simulink model "VSCHVDCunitblackstart"  (R2025b)
settings: Solver=VariableStepAuto  StartTime=0  StopTime=25  FixedStep=5e-5  RelTol=1e-3
PreLoadFcn:
  | HVDCParameters;
  | BlackStartMMCParameters;
undefined symbols (not defined in the file): DiscIntNeverNeededParam, FRated, frt, gGFM, grid, Lbase, Lr, Lt, lvrt, mGFM, mpptOmega, mpptWindSpeed, Nm, pmsm, PRated, Rc, rpir, Rr, Rt, time, Tpir, Ts, Vbase, Vdcs0, VRated, Vt2, windController, windTurbine, Zbase
libraries: fl_lib x47, ee_lib x41, nesl_utility x33, eeGeneralControl x13, eeTransforms x12, slpidlib x8, eeSinusoidalMeasurementV2 x4, simulink x2, eeSinusoidalMeasurement x1, eeStairGenerator x1
(part 1 of 5)
settings Model: SimulationMode=accelerator  Creator=Rajarshi  LastModifiedBy=rajarshd
settings SolverCC: ZeroCrossControl=DisableAll  ZeroCrossAlgorithm=Adaptive  AutoInsertRateTranBlk=on
settings DataIOCC: InitialState=xFinal  SaveFormat=StructureWithTime  SaveOutput=off  DSMLogging=off  StreamToWks=off  SaveTime=off  ReturnWorkspaceOutputsName=blackstartResults
settings DebuggingCC: InheritedTsInSrcMsg=none
settings ModelReferenceCC: PropagateSignalLabelsOutOfModel=off
settings SimscapeCC: SimscapeNormalizeSystem=off

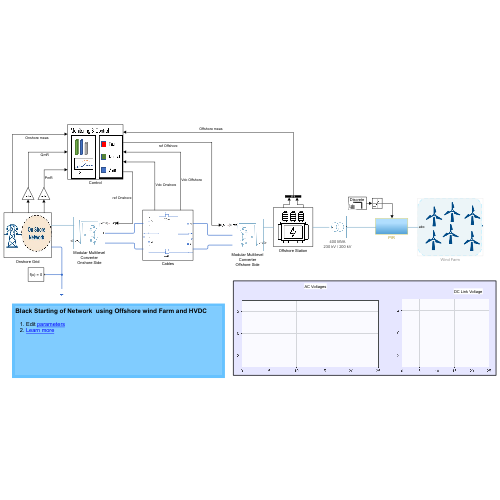
[thumbnail: Simulink's stored preview of the top-level diagram]
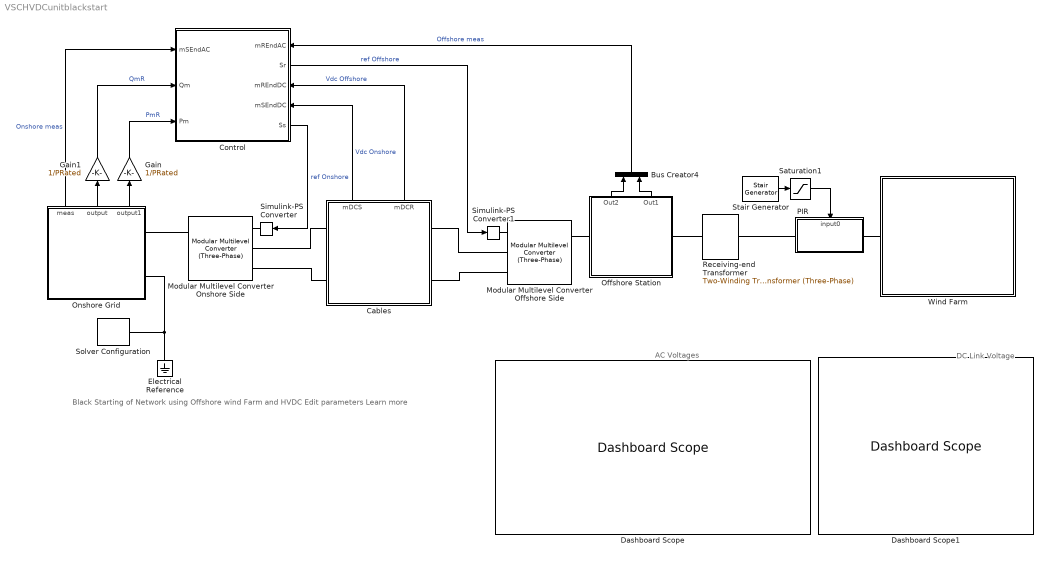
== system VSCHVDCunitblackstart ==
  note: DC Link Voltage
  note: AC Voltages
  note: Black Starting of Network using Offshore wind Farm and HVDC
      |
      | Edit parameters
      | Learn more
  Bus Creator4 : BusCreator  Inputs=2
  Cables : Subsystem
      settings: PortSchema="{\"entries\":[{\"content\":{\"sides\":[{\"content\":{\"connectorIds\":[\"LConn1\",\"LConn2\"]},\"type\":\"ConnectorPlacement.EquallySpacedRectSide\",\"uuid\":\"66d4cfbf-dcba-4749-bf5d-5811a775276e\"},{\"content\":{\"connectorIds\":[\"RConn1\",\"RConn2\"],\"side\":\"RIGHT\"},\"type\":\"ConnectorPlacement.EquallySpacedRectSide\",\"uuid\":\"35abdffa-cda0-46f2-9903-3f86a9532248\"},{\"content\":{\"connectorIds\":[\"Out1\",\"Out2\"],\"side\":\"TOP\"},\"type\":\"ConnectorPlacement.EquallySpacedRectSide\",\"uuid\":\"3c5502e5-1b76-444d-b26b-a5789383a319\"}]},\"type\":\"ConnectorPlacement.EquallySpacedConnector\",\"uuid\":\"b78b2c4f-7eb3-43f3-aa61-891430661a3a\"}],\"packageUris\":[\"http://schema.mathworks.com/mf0/Connector/R2020b\"],\"version\":\"1.0\"}"
      mask Display: image('HVDCCable.PNG');
  Control : Subsystem
      settings: PortSchema="{\"entries\":[{\"content\":{\"sides\":[{\"content\":{\"connectorIds\":[\"In1\",\"In2\",\"In3\"]},\"type\":\"ConnectorPlacement.EquallySpacedRectSide\",\"uuid\":\"2efe798b-3041-46d6-be94-ed23c5e86f39\"},{\"content\":{\"connectorIds\":[\"In4\",\"Out1\",\"In5\",\"In6\",\"Out2\"],\"side\":\"RIGHT\"},\"type\":\"ConnectorPlacement.EquallySpacedRectSide\",\"uuid\":\"10311844-b4ae-4332-a927-ed09106eeb00\"},{\"content\":{\"side\":\"TOP\"},\"type\":\"ConnectorPlacement.EquallySpacedRectSide\",\"uuid\":\"46c0cb94-5d38-4b98-8b78-a07f64b43f47\"}]},\"type\":\"ConnectorPlacement.EquallySpacedConnector\",\"uuid\":\"cfce9429-7807-479b-aecd-c199f821abc4\"}],\"packageUris\":[\"http://schema.mathworks.com/mf0/Connector/R2020b\"],\"version\":\"1.0\"}"
      mask Display: image('Contol_room.png');
  Dashboard Scope : DashboardScope  FontColor=[0.0, 0.0, 0.0]
  Dashboard Scope1 : DashboardScope  FontColor=[0.0, 0.0, 0.0]
  Electrical Reference : fl_lib/Electrical/Electrical Elements/Electrical Reference
  Gain : Gain  Gain=1/PRated
  Gain1 : Gain  Gain=1/PRated
  Modular Multilevel Converter Offshore Side : ee_lib/Semiconductors & Converters/Converters/Modular Multilevel Converter (Three-Phase)  port_option=ee.enum.threePhasePort.composite  topology_option=ee.enum.converters.mmctopology.halfbridge  fidelity_option=ee.enum.converters.mmcfidelity.equivalent_waveform  meas_option=ee.enum.internalvariables.instrumented  Nsm=4  Csm=Cm F  Rsm=1e-6 Ohm  La=1e-6 H  Ra=0 Ohm  vc_init=0 V  device_type=ee.enum.converters.switchingdevice.ideal  K=0  Vf=0.8 V  Ron=0.001 Ohm  Rds=0.001 Ohm  Goff=1e-5 1/Ohm  Vgt=1 V  Vgt_off=-1 V  Ih=1 A  Vth=6 V  diode_param=ee.enum.converters.protectiondiode.nodynamics  diode_Vf=0.8 V  diode_Ron=0.001 Ohm  diode_Goff=1e-5 1/Ohm  diode_C=50 nF  diode_iRM=-235 A  diode_iF=300 A  diode_idot=-50 A/us  diode_trr_param=ee.enum.converters.diodetrr.trr_factor  diode_trr_factor=3  diode_trr=15 us  diode_Qrr=1500 s*uA  snubber_type=ee.enum.converters.snubber.exclude  Cs=1e-7 F  Rs=0.1 Ohm  iLpa_specify=off  iLpa_priority=None  iLpa=0 A  iLpa_nominal_specify=off  iLpa_nominal_value=1  iLpa_nominal_unit=A  iLna_specify=off  iLna_priority=None  iLna=0 A  iLna_nominal_specify=off  iLna_nominal_value=1  iLna_nominal_unit=A  iLpb_specify=off  iLpb_priority=None  iLpb=0 A  iLpb_nominal_specify=off  iLpb_nominal_value=1  iLpb_nominal_unit=A  iLnb_specify=off  iLnb_priority=None  iLnb=0 A  iLnb_nominal_specify=off  iLnb_nominal_value=1  iLnb_nominal_unit=A  iLpc_specify=off  iLpc_priority=None  iLpc=0 A  iLpc_nominal_specify=off  iLpc_nominal_value=1  iLpc_nominal_unit=A  iLnc_specify=off  iLnc_priority=None  iLnc=0 A  iLnc_nominal_specify=off  iLnc_nominal_value=1  iLnc_nominal_unit=A
      settings: InternalSimscapePortConfiguration="{\"Bottom\":[],\"Left\":[{\"id\":\"ref\",\"label\":\"ref\",\"type\":\"input\"},{\"id\":\"p\",\"label\":\"+\",\"type\":\"foundation.electrical.electrical\"},{\"id\":\"n\",\"label\":\"-\",\"type\":\"foundation.electrical.electrical\"}],\"Right\":[{\"id\":\"N\",\"label\":\"~\",\"type\":\"foundation.electrical.three_phase\"},{\"id\":\"vc_out\",\"label\":\"vc\",\"type\":\"output\"}],\"Top\":[]}"
  Modular Multilevel Converter Onshore Side : ee_lib/Semiconductors & Converters/Converters/Modular Multilevel Converter (Three-Phase)  port_option=ee.enum.threePhasePort.composite  topology_option=ee.enum.converters.mmctopology.halfbridge  fidelity_option=ee.enum.converters.mmcfidelity.equivalent_waveform  meas_option=ee.enum.internalvariables.instrumented  Nsm=4  Csm=Cm F  Rsm=1e-6 Ohm  La=1e-6 H  Ra=0 Ohm  vc_init=0 V  device_type=ee.enum.converters.switchingdevice.ideal  K=0  Vf=0.8 V  Ron=0.001 Ohm  Rds=0.001 Ohm  Goff=1e-5 1/Ohm  Vgt=1 V  Vgt_off=-1 V  Ih=1 A  Vth=6 V  diode_param=ee.enum.converters.protectiondiode.nodynamics  diode_Vf=0.8 V  diode_Ron=0.001 Ohm  diode_Goff=1e-5 1/Ohm  diode_C=50 nF  diode_iRM=-235 A  diode_iF=300 A  diode_idot=-50 A/us  diode_trr_param=ee.enum.converters.diodetrr.trr_factor  diode_trr_factor=3  diode_trr=15 us  diode_Qrr=1500 s*uA  snubber_type=ee.enum.converters.snubber.exclude  Cs=1e-7 F  Rs=0.1 Ohm  iLpa_specify=off  iLpa_priority=None  iLpa=0 A  iLpa_nominal_specify=off  iLpa_nominal_value=1  iLpa_nominal_unit=A  iLna_specify=off  iLna_priority=None  iLna=0 A  iLna_nominal_specify=off  iLna_nominal_value=1  iLna_nominal_unit=A  iLpb_specify=off  iLpb_priority=None  iLpb=0 A  iLpb_nominal_specify=off  iLpb_nominal_value=1  iLpb_nominal_unit=A  iLnb_specify=off  iLnb_priority=None  iLnb=0 A  iLnb_nominal_specify=off  iLnb_nominal_value=1  iLnb_nominal_unit=A  iLpc_specify=off  iLpc_priority=None  iLpc=0 A  iLpc_nominal_specify=off  iLpc_nominal_value=1  iLpc_nominal_unit=A  iLnc_specify=off  iLnc_priority=None  iLnc=0 A  iLnc_nominal_specify=off  iLnc_nominal_value=1  iLnc_nominal_unit=A
      settings: InternalSimscapePortConfiguration="{\"Bottom\":[],\"Left\":[{\"id\":\"ref\",\"label\":\"ref\",\"type\":\"input\"},{\"id\":\"p\",\"label\":\"+\",\"type\":\"foundation.electrical.electrical\"},{\"id\":\"n\",\"label\":\"-\",\"type\":\"foundation.electrical.electrical\"}],\"Right\":[{\"id\":\"N\",\"label\":\"~\",\"type\":\"foundation.electrical.three_phase\"},{\"id\":\"vc_out\",\"label\":\"vc\",\"type\":\"output\"}],\"Top\":[]}"
  Offshore Station : Subsystem
      settings: PortSchema="{\"entries\":[{\"content\":{\"sides\":[{\"content\":{\"connectorIds\":[\"LConn1\"]},\"type\":\"ConnectorPlacement.EquallySpacedRectSide\",\"uuid\":\"33871510-c6a2-4027-b2f7-c1a24bc72d9b\"},{\"content\":{\"connectorIds\":[\"RConn1\"],\"side\":\"RIGHT\"},\"type\":\"ConnectorPlacement.EquallySpacedRectSide\",\"uuid\":\"4190d4bc-8e21-4e1a-b664-4821c6e49c1e\"},{\"content\":{\"connectorIds\":[\"Out1\",\"Out2\"],\"side\":\"TOP\"},\"type\":\"ConnectorPlacement.EquallySpacedRectSide\",\"uuid\":\"d8f10822-ee6b-47b4-9885-677b57914fd5\"}]},\"type\":\"ConnectorPlacement.EquallySpacedConnector\",\"uuid\":\"45fab97f-4e1a-4d80-a844-d46aeb4cf0fc\"}],\"packageUris\":[\"http://schema.mathworks.com/mf0/Connector/R2020b\"],\"version\":\"1.0\"}"
      mask Display: image('transformer.png');
  Onshore Grid : Subsystem
      settings: PortSchema="{\"entries\":[{\"content\":{\"sides\":[{\"content\":{},\"type\":\"ConnectorPlacement.EquallySpacedRectSide\",\"uuid\":\"33871510-c6a2-4027-b2f7-c1a24bc72d9b\"},{\"content\":{\"connectorIds\":[\"RConn1\",\"RConn2\"],\"side\":\"RIGHT\"},\"type\":\"ConnectorPlacement.EquallySpacedRectSide\",\"uuid\":\"4190d4bc-8e21-4e1a-b664-4821c6e49c1e\"},{\"content\":{\"connectorIds\":[\"Out1\",\"Out2\",\"Out3\"],\"side\":\"TOP\"},\"type\":\"ConnectorPlacement.EquallySpacedRectSide\",\"uuid\":\"d8f10822-ee6b-47b4-9885-677b57914fd5\"},{\"content\":{\"side\":\"BOTTOM\"},\"type\":\"ConnectorPlacement.EquallySpacedRectSide\",\"uuid\":\"afe5fd03-9d9a-430d-816a-6986d2bc632f\"}]},\"type\":\"ConnectorPlacement.EquallySpacedConnector\",\"uuid\":\"45fab97f-4e1a-4d80-a844-d46aeb4cf0fc\"}],\"packageUris\":[\"http://schema.mathworks.com/mf0/Connector/R2020b\"],\"version\":\"1.0\"}"
      mask Display: image('onshoreNetwork.jpg');
  PIR : Subsystem
      settings: PortSchema="{\"entries\":[{\"content\":{\"sides\":[{\"content\":{\"connectorIds\":[\"LConn1\"]},\"type\":\"ConnectorPlacement.EquallySpacedRectSide\",\"uuid\":\"67c0f727-7c15-41c9-98df-b3c7d57498ed\"},{\"content\":{\"connectorIds\":[\"RConn1\"],\"side\":\"RIGHT\"},\"type\":\"ConnectorPlacement.EquallySpacedRectSide\",\"uuid\":\"7fc39429-ba61-416d-b42b-93e81eb2f426\"},{\"content\":{\"side\":\"TOP\"},\"type\":\"ConnectorPlacement.EquallySpacedRectSide\",\"uuid\":\"c6dd9263-b57a-4cff-a218-af99f2798f29\"},{\"content\":{\"connectorIds\":[\"In1\"],\"side\":\"BOTTOM\"},\"type\":\"ConnectorPlacement.EquallySpacedRectSide\",\"uuid\":\"e2a2ba44-d59d-4e27-adf1-3f94e828ca78\"}]},\"type\":\"ConnectorPlacement.EquallySpacedConnector\",\"uuid\":\"b349a99b-c902-4df9-9c99-34841afb28dd\"}],\"packageUris\":[\"http://schema.mathworks.com/mf0/Connector/R2020b\"],\"version\":\"1.0\"}"
  Receiving-end Transformer : ee_lib/Passive/Transformers/Two-Winding Transformer (Three-Phase)  SRated=Pnom A*V  FRated=FRated Hz  Winding1Connection=ee.enum.windingconnection.Yg  VRated1=4.16e3 V  Winding2Connection=ee.enum.windingconnection.Yg  VRated2=230e3 V  CoreType=ee.enum.coretype.fivelimb  pu_Rw1=1e-3  pu_Rw2=1e-3  leakage_reactance_option=ee.enum.transformer_leakage.include  pu_Xl1=0.01  pu_Xl2=0.01  magnetizing_resistance_option=ee.enum.transformer_magnetizingResistance.include  pu_Rm=500  magnetizing_reactance_option=ee.enum.transformer_magnetizingReactance.include  saturation_option=ee.enum.transformer_saturation.exclude  pu_Xm=500  current_data=[0, .002, 1, 2]  magnetic_flux_data=[0, 1.2, 1.5, 1.51]  pu_X0=0.5  i1_specify=off  i1_priority=None  i1=[0, 0, 0] A  i1_nominal_specify=off  i1_nominal_value=1  i1_nominal_unit=A  i2_specify=off  i2_priority=None  i2=[0, 0, 0] A  i2_nominal_specify=off  i2_nominal_value=1  i2_nominal_unit=A  phi_specify=off  phi_priority=None  phi=[0, 0, 0]  phi_nominal_specify=off  phi_nominal_value=1  phi_nominal_unit=1  power_dissipated_specify=off  power_dissipated_priority=None  power_dissipated=0 W  power_dissipated_nominal_specify=off  power_dissipated_nominal_value=1  power_dissipated_nominal_unit=W
      settings: InternalSimscapePortConfiguration="{\"Bottom\":[],\"Left\":[{\"id\":\"N1\",\"label\":\"~1\",\"type\":\"foundation.electrical.three_phase\"}],\"Right\":[{\"id\":\"N2\",\"label\":\"~2\",\"type\":\"foundation.electrical.three_phase\"}],\"Top\":[]}"
      settings: AttributesFormatString=|
      | 400 MVA
      | 230 kV / 200 kV
  Saturation1 : Saturate  UpperLimit=1  LowerLimit=0
  Simulink-PS Converter : nesl_utility/Simulink-PS Converter  PhysicalDomain=network_engine_domain  SubClassName=ps_input  LeftPortType=input  RightPortType=output  PseudoPeriodic=off  Frequencies=[]  NoiseDistribution=none  NoiseParameters=[]  Unit=1  AffineConversion=off  FilteringAndDerivatives=provide  SimscapeFilterOrder=1  InputFilterTimeConstant=0.001  UdotUserProvided=0
  Simulink-PS Converter1 : nesl_utility/Simulink-PS Converter  PhysicalDomain=network_engine_domain  SubClassName=ps_input  LeftPortType=input  RightPortType=output  PseudoPeriodic=off  Frequencies=[]  NoiseDistribution=none  NoiseParameters=[]  Unit=1  AffineConversion=off  FilteringAndDerivatives=provide  SimscapeFilterOrder=1  InputFilterTimeConstant=0.001  UdotUserProvided=0
  Solver Configuration : nesl_utility/Solver Configuration  PhysicalDomain=network_engine_domain  SubClassName=solver  LeftPortType=input  RightPortType=generic  Tones=[]  Harmonics=[]  SimulateNoise=off  Profile=off  UseLocalSampling=off  EnableSwitchedLinearOptims=on  FrequencyDomain=off  UseCCode=off  RelTol=0.001  AbsTol=0.001  MinStep=1e-09  ToWorkspace=off  RevertToSquareIcSolve=off  NumHomotopyIterations=100  PhasorMode=off  PhasorModeNumHarmonics=1  ConsistencySolver=NEWTON_XTOL_AFTER_FTOL  IndexReductionMethod=None  DoDC=off  ResidualTolerance=1e-09  ConsistencyTolSource=GLOBAL  ConsistencyAbsTol=1e5  ConsistencyRelTol=1e5  ConsistencyTolFactor=1e3  UseLocalSolver=on  LocalSolverChoice=NE_BACKWARD_EULER_ADVANCER  ResolveIndetEquations=off  FunctionEvalNumThread=1  LocalSolverSampleTime=Ts*6  DoFixedCost=on  MaxNonlinIter=3  MaxModeIter=2  ComputeImpulses=off  ImpulseIterations=2  LinearAlgebra=Sparse  LinearAlgebraNumThread=0  EquationFormulation=NE_TIME_EF  DelaysMemoryBudget=1024  AutomaticFiltering=off  FilteringTimeConstant=0.001  PartitionStorageMethod=AS_NEEDED  PartitionMemoryBudget=1024  PartitionMethod=ROBUST  MultibodyUseLocalSolver=off  MultibodyLocalSolverChoice=ODE1  MultibodyLocalSolverSampleTime=0.001
  Stair Generator : eeStairGenerator/Stair Generator  LabelModeActiveChoice=Discrete  TimeInput=[0 Tpir]  AmplitudeInput=[rpir 0]  SampleTime=-1  RepeatPattern=off  OutDataTypeStr=double
      settings: LibrarySourceBlock=ee_sl_lib/General Control/Stair Generator
  Wind Farm : Subsystem
      mask Display: image('windFarmOff.PNG');
  wires:
  Cables/2(mDCR) -> Control/5(mREndDC)  "Vdc Offshore"
  Stair Generator/1 -> Saturation1/1
  Onshore Grid/3(output1) -> Gain/1
  Offshore Station/1(Out1) -> Bus Creator4/2
  Control/2(Ss) -> Simulink-PS Converter/1  "ref Onshore"
  Saturation1/1 -> PIR/1(input0)
  Onshore Grid/1(meas) -> Control/1(mSEndAC)  "Onshore meas"
  Control/1(Sr) -> Simulink-PS Converter1/1  "ref Offshore"
  Cables/1(mDCS) -> Control/6(mSEndDC)  "Vdc Onshore"
  Gain1/1 -> Control/2(Qm)  "QmR"
  Onshore Grid/2(output) -> Gain1/1
  Gain/1 -> Control/3(Pm)  "PmR"
  Bus Creator4/1 -> Control/4(mREndAC)  "Offshore meas"
  Offshore Station/2(Out2) -> Bus Creator4/1
  connections:
  Simulink-PS Converter1/RConn1 -- Modular Multilevel Converter Offshore Side/LConn1
  Cables/RConn1 -- Modular Multilevel Converter Offshore Side/LConn2
  Modular Multilevel Converter Onshore Side/LConn2 -- Cables/LConn1
  Modular Multilevel Converter Onshore Side/LConn3 -- Cables/LConn2
  Cables/RConn2 -- Modular Multilevel Converter Offshore Side/LConn3
  Simulink-PS Converter/RConn1 -- Modular Multilevel Converter Onshore Side/LConn1
  Electrical Reference/LConn1 -- Solver Configuration/RConn1 -- Onshore Grid/RConn2
  Modular Multilevel Converter Onshore Side/RConn1 -- Onshore Grid/RConn1
  Modular Multilevel Converter Offshore Side/RConn1 -- Offshore Station/RConn1
  Wind Farm/RConn1 -- PIR/RConn1
  Receiving-end Transformer/RConn1 -- Offshore Station/LConn1
  Receiving-end Transformer/LConn1 -- PIR/LConn1

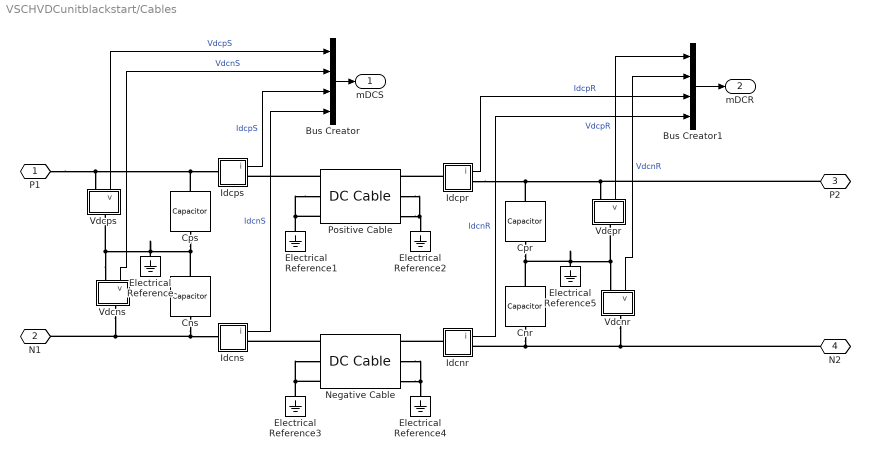
== system VSCHVDCunitblackstart/Cables ==
  Bus Creator : BusCreator  Inputs=4
  Bus Creator1 : BusCreator  Inputs=4
  Cnr : fl_lib/Electrical/Electrical Elements/Capacitor  c=Cdc F  r=Rdc Ohm  g=0 1/Ohm  i_specify=off  i_priority=High  i=0 A  i_nominal_specify=off  i_nominal_value=1  i_nominal_unit=A  v_specify=off  v_priority=High  v=Vdcs0/2 V  v_nominal_specify=off  v_nominal_value=1  v_nominal_unit=V  vc_specify=on  vc_priority=None  vc=0 V  vc_nominal_specify=off  vc_nominal_value=1  vc_nominal_unit=V
  Cns : fl_lib/Electrical/Electrical Elements/Capacitor  c=Cdc F  r=Rdc Ohm  g=0 1/Ohm  i_specify=off  i_priority=High  i=0 A  i_nominal_specify=off  i_nominal_value=1  i_nominal_unit=A  v_specify=off  v_priority=High  v=Vdcs0/2 V  v_nominal_specify=off  v_nominal_value=1  v_nominal_unit=V  vc_specify=on  vc_priority=None  vc=1e-1 V  vc_nominal_specify=off  vc_nominal_value=1  vc_nominal_unit=V
  Cpr : fl_lib/Electrical/Electrical Elements/Capacitor  c=Cdc F  r=Rdc Ohm  g=0 1/Ohm  i_specify=off  i_priority=High  i=0 A  i_nominal_specify=off  i_nominal_value=1  i_nominal_unit=A  v_specify=off  v_priority=High  v=Vdcs0/2 V  v_nominal_specify=off  v_nominal_value=1  v_nominal_unit=V  vc_specify=on  vc_priority=None  vc=0 V  vc_nominal_specify=off  vc_nominal_value=1  vc_nominal_unit=V
  Cps : fl_lib/Electrical/Electrical Elements/Capacitor  c=Cdc F  r=Rdc Ohm  g=0 1/Ohm  i_specify=off  i_priority=High  i=0 A  i_nominal_specify=off  i_nominal_value=1  i_nominal_unit=A  v_specify=off  v_priority=High  v=Vdcs0/2 V  v_nominal_specify=off  v_nominal_value=1  v_nominal_unit=V  vc_specify=on  vc_priority=None  vc=1e-1 V  vc_nominal_specify=off  vc_nominal_value=1  vc_nominal_unit=V
  Electrical Reference{,1..5} (6 alike) : fl_lib/Electrical/Electrical Elements/Electrical Reference
  Idcnr : Subsystem
      settings: PortSchema="{\"entries\":[{\"content\":{\"sides\":[{\"content\":{\"connectorIds\":[\"LConn1\"]},\"type\":\"ConnectorPlacement.EquallySpacedRectSide\",\"uuid\":\"b182dbc5-c8d5-4832-a7cd-ea3787954646\"},{\"content\":{\"connectorIds\":[\"RConn1\",\"Out1\"],\"side\":\"RIGHT\"},\"type\":\"ConnectorPlacement.EquallySpacedRectSide\",\"uuid\":\"bfc6f163-1abf-440b-aa89-1443f971fd07\"},{\"content\":{\"connectorIds\":[],\"side\":\"TOP\"},\"type\":\"ConnectorPlacement.EquallySpacedRectSide\",\"uuid\":\"dd2a104c-9a72-483e-91c4-dbef9b359450\"}]},\"type\":\"ConnectorPlacement.EquallySpacedConnector\",\"uuid\":\"ce98cc3b-f524-409d-a465-fff2e3b7df79\"}],\"packageUris\":[\"http://schema.mathworks.com/mf0/Connector/R2020b\"],\"version\":\"1.0\"}"
  Idcns : Subsystem
      settings: PortSchema="{\"entries\":[{\"content\":{\"sides\":[{\"content\":{\"connectorIds\":[\"LConn1\"]},\"type\":\"ConnectorPlacement.EquallySpacedRectSide\",\"uuid\":\"b182dbc5-c8d5-4832-a7cd-ea3787954646\"},{\"content\":{\"connectorIds\":[\"RConn1\",\"Out1\"],\"side\":\"RIGHT\"},\"type\":\"ConnectorPlacement.EquallySpacedRectSide\",\"uuid\":\"bfc6f163-1abf-440b-aa89-1443f971fd07\"},{\"content\":{\"connectorIds\":[],\"side\":\"TOP\"},\"type\":\"ConnectorPlacement.EquallySpacedRectSide\",\"uuid\":\"dd2a104c-9a72-483e-91c4-dbef9b359450\"}]},\"type\":\"ConnectorPlacement.EquallySpacedConnector\",\"uuid\":\"ce98cc3b-f524-409d-a465-fff2e3b7df79\"}],\"packageUris\":[\"http://schema.mathworks.com/mf0/Connector/R2020b\"],\"version\":\"1.0\"}"
  Idcpr : Subsystem
      settings: PortSchema="{\"entries\":[{\"content\":{\"sides\":[{\"content\":{\"connectorIds\":[\"LConn1\"]},\"type\":\"ConnectorPlacement.EquallySpacedRectSide\",\"uuid\":\"b182dbc5-c8d5-4832-a7cd-ea3787954646\"},{\"content\":{\"connectorIds\":[\"RConn1\",\"Out1\"],\"side\":\"RIGHT\"},\"type\":\"ConnectorPlacement.EquallySpacedRectSide\",\"uuid\":\"bfc6f163-1abf-440b-aa89-1443f971fd07\"},{\"content\":{\"connectorIds\":[],\"side\":\"TOP\"},\"type\":\"ConnectorPlacement.EquallySpacedRectSide\",\"uuid\":\"dd2a104c-9a72-483e-91c4-dbef9b359450\"}]},\"type\":\"ConnectorPlacement.EquallySpacedConnector\",\"uuid\":\"ce98cc3b-f524-409d-a465-fff2e3b7df79\"}],\"packageUris\":[\"http://schema.mathworks.com/mf0/Connector/R2020b\"],\"version\":\"1.0\"}"
  Idcps : Subsystem
      settings: PortSchema="{\"entries\":[{\"content\":{\"sides\":[{\"content\":{\"connectorIds\":[\"LConn1\"]},\"type\":\"ConnectorPlacement.EquallySpacedRectSide\",\"uuid\":\"b182dbc5-c8d5-4832-a7cd-ea3787954646\"},{\"content\":{\"connectorIds\":[\"RConn1\",\"Out1\"],\"side\":\"RIGHT\"},\"type\":\"ConnectorPlacement.EquallySpacedRectSide\",\"uuid\":\"bfc6f163-1abf-440b-aa89-1443f971fd07\"},{\"content\":{\"connectorIds\":[],\"side\":\"TOP\"},\"type\":\"ConnectorPlacement.EquallySpacedRectSide\",\"uuid\":\"dd2a104c-9a72-483e-91c4-dbef9b359450\"}]},\"type\":\"ConnectorPlacement.EquallySpacedConnector\",\"uuid\":\"ce98cc3b-f524-409d-a465-fff2e3b7df79\"}],\"packageUris\":[\"http://schema.mathworks.com/mf0/Connector/R2020b\"],\"version\":\"1.0\"}"
  Negative Cable : ee_lib/Passive/Lines/DC Cable  configuration_option=ee.enum.powerCable.dc_configuration.one  rho_env=100 Ohm*m  len=85 km  rho_c=2.1e-8 Ohm*m  mur_c=1  mur_i=1  epsilon_i=2.5  rho_sh=2.2e-7 Ohm*m  mur_sh=1  mur_j=1  epsilon_j=2.4  rho_a=1.8e-7 Ohm*m  mur_a=10  mur_se=1  epsilon_se=2.4  rth_c=25 mm  rth_i=20 mm  rth_sh=3 mm  rth_j=5 mm  rth_a=6 mm  rth_se=5 mm  pos_single_y=1 m  pos_double_y=[1, 1] m  pos_double_x=[0, 1] m  Vp_specify=off  Vp_priority=High  Vp=[0, 0, 0] V  Vp_nominal_specify=off  Vp_nominal_value=1  Vp_nominal_unit=V  Vn_specify=off  Vn_priority=High  Vn=[0, 0, 0] V  Vn_nominal_specify=off  Vn_nominal_value=1  Vn_nominal_unit=V  Ip_specify=off  Ip_priority=High  Ip=[0, 0, 0] A  Ip_nominal_specify=off  Ip_nominal_value=1  Ip_nominal_unit=A  In_specify=off  In_priority=High  In=[0, 0, 0] A  In_nominal_specify=off  In_nominal_value=1  In_nominal_unit=A  V1p_specify=off  V1p_priority=None  V1p=[0, 0, 0] V  V1p_nominal_specify=off  V1p_nominal_value=1  V1p_nominal_unit=V  V1n_specify=off  V1n_priority=None  V1n=[0, 0, 0] V  V1n_nominal_specify=off  V1n_nominal_value=1  V1n_nominal_unit=V  I1p_specify=off  I1p_priority=None  I1p=[0, 0, 0] A  I1p_nominal_specify=off  I1p_nominal_value=1  I1p_nominal_unit=A  I1n_specify=off  I1n_priority=None  I1n=[0, 0, 0] A  I1n_nominal_specify=off  I1n_nominal_value=1  I1n_nominal_unit=A  V2p_specify=off  V2p_priority=None  V2p=[0, 0, 0] V  V2p_nominal_specify=off  V2p_nominal_value=1  V2p_nominal_unit=V  V2n_specify=off  V2n_priority=None  V2n=[0, 0, 0] V  V2n_nominal_specify=off  V2n_nominal_value=1  V2n_nominal_unit=V  I2p_specify=off  I2p_priority=None  I2p=[0, 0, 0] A  I2p_nominal_specify=off  I2p_nominal_value=1  I2p_nominal_unit=A  I2n_specify=off  I2n_priority=None  I2n=[0, 0, 0] A  I2n_nominal_specify=off  I2n_nominal_value=1  I2n_nominal_unit=A
      settings: InternalSimscapePortConfiguration="{\"Bottom\":[],\"Left\":[{\"id\":\"cp\",\"label\":\"c+\",\"type\":\"foundation.electrical.electrical\"},{\"id\":\"sp\",\"label\":\"s+\",\"type\":\"foundation.electrical.electrical\"},{\"id\":\"ap\",\"label\":\"a+\",\"type\":\"foundation.electrical.electrical\"}],\"Right\":[{\"id\":\"cn\",\"label\":\"c-\",\"type\":\"foundation.electrical.electrical\"},{\"id\":\"sn\",\"label\":\"s-\",\"type\":\"foundation.electrical.electrical\"},{\"id\":\"an\",\"label\":\"a-\",\"type\":\"foundation.electrical.electrical\"}],\"Top\":[]}"
  Positive Cable : ee_lib/Passive/Lines/DC Cable  configuration_option=ee.enum.powerCable.dc_configuration.one  rho_env=100 Ohm*m  len=85 km  rho_c=2.1e-8 Ohm*m  mur_c=1  mur_i=1  epsilon_i=2.5  rho_sh=2.2e-7 Ohm*m  mur_sh=1  mur_j=1  epsilon_j=2.4  rho_a=1.8e-7 Ohm*m  mur_a=10  mur_se=1  epsilon_se=2.4  rth_c=25 mm  rth_i=20 mm  rth_sh=3 mm  rth_j=5 mm  rth_a=6 mm  rth_se=5 mm  pos_single_y=1 m  pos_double_y=[1, 1] m  pos_double_x=[0, 1] m  Vp_specify=off  Vp_priority=High  Vp=[0, 0, 0] V  Vp_nominal_specify=off  Vp_nominal_value=1  Vp_nominal_unit=V  Vn_specify=off  Vn_priority=High  Vn=[0, 0, 0] V  Vn_nominal_specify=off  Vn_nominal_value=1  Vn_nominal_unit=V  Ip_specify=off  Ip_priority=High  Ip=[0, 0, 0] A  Ip_nominal_specify=off  Ip_nominal_value=1  Ip_nominal_unit=A  In_specify=off  In_priority=High  In=[0, 0, 0] A  In_nominal_specify=off  In_nominal_value=1  In_nominal_unit=A  V1p_specify=off  V1p_priority=None  V1p=[0, 0, 0] V  V1p_nominal_specify=off  V1p_nominal_value=1  V1p_nominal_unit=V  V1n_specify=off  V1n_priority=None  V1n=[0, 0, 0] V  V1n_nominal_specify=off  V1n_nominal_value=1  V1n_nominal_unit=V  I1p_specify=off  I1p_priority=None  I1p=[0, 0, 0] A  I1p_nominal_specify=off  I1p_nominal_value=1  I1p_nominal_unit=A  I1n_specify=off  I1n_priority=None  I1n=[0, 0, 0] A  I1n_nominal_specify=off  I1n_nominal_value=1  I1n_nominal_unit=A  V2p_specify=off  V2p_priority=None  V2p=[0, 0, 0] V  V2p_nominal_specify=off  V2p_nominal_value=1  V2p_nominal_unit=V  V2n_specify=off  V2n_priority=None  V2n=[0, 0, 0] V  V2n_nominal_specify=off  V2n_nominal_value=1  V2n_nominal_unit=V  I2p_specify=off  I2p_priority=None  I2p=[0, 0, 0] A  I2p_nominal_specify=off  I2p_nominal_value=1  I2p_nominal_unit=A  I2n_specify=off  I2n_priority=None  I2n=[0, 0, 0] A  I2n_nominal_specify=off  I2n_nominal_value=1  I2n_nominal_unit=A
      settings: InternalSimscapePortConfiguration="{\"Bottom\":[],\"Left\":[{\"id\":\"cp\",\"label\":\"c+\",\"type\":\"foundation.electrical.electrical\"},{\"id\":\"sp\",\"label\":\"s+\",\"type\":\"foundation.electrical.electrical\"},{\"id\":\"ap\",\"label\":\"a+\",\"type\":\"foundation.electrical.electrical\"}],\"Right\":[{\"id\":\"cn\",\"label\":\"c-\",\"type\":\"foundation.electrical.electrical\"},{\"id\":\"sn\",\"label\":\"s-\",\"type\":\"foundation.electrical.electrical\"},{\"id\":\"an\",\"label\":\"a-\",\"type\":\"foundation.electrical.electrical\"}],\"Top\":[]}"
  Vdcnr : Subsystem
      settings: PortSchema="{\"entries\":[{\"content\":{\"sides\":[{\"content\":{\"connectorIds\":[\"LConn1\",\"Out1\"]},\"type\":\"ConnectorPlacement.EquallySpacedRectSide\",\"uuid\":\"bc3757cc-4537-444e-89af-7b7d8c8c1fa7\"},{\"content\":{\"connectorIds\":[\"RConn1\"],\"side\":\"RIGHT\"},\"type\":\"ConnectorPlacement.EquallySpacedRectSide\",\"uuid\":\"908bf4c4-26f6-4d8a-bcf8-68236027f5f8\"},{\"content\":{\"side\":\"TOP\"},\"type\":\"ConnectorPlacement.EquallySpacedRectSide\",\"uuid\":\"33f228db-ba47-4718-96dc-a72de309ae8c\"},{\"content\":{\"side\":\"BOTTOM\"},\"type\":\"ConnectorPlacement.EquallySpacedRectSide\",\"uuid\":\"d9b66c7e-0954-4c47-8bcc-77bf13ff573c\"}]},\"type\":\"ConnectorPlacement.EquallySpacedConnector\",\"uuid\":\"345f3578-0572-4e64-b2f3-84728129a12d\"}],\"packageUris\":[\"http://schema.mathworks.com/mf0/Connector/R2020b\"],\"version\":\"1.0\"}"
  Vdcns : Subsystem
      settings: PortSchema="{\"entries\":[{\"content\":{\"sides\":[{\"content\":{\"connectorIds\":[\"LConn1\",\"Out1\"]},\"type\":\"ConnectorPlacement.EquallySpacedRectSide\",\"uuid\":\"bc3757cc-4537-444e-89af-7b7d8c8c1fa7\"},{\"content\":{\"connectorIds\":[\"RConn1\"],\"side\":\"RIGHT\"},\"type\":\"ConnectorPlacement.EquallySpacedRectSide\",\"uuid\":\"908bf4c4-26f6-4d8a-bcf8-68236027f5f8\"},{\"content\":{\"side\":\"TOP\"},\"type\":\"ConnectorPlacement.EquallySpacedRectSide\",\"uuid\":\"33f228db-ba47-4718-96dc-a72de309ae8c\"},{\"content\":{\"side\":\"BOTTOM\"},\"type\":\"ConnectorPlacement.EquallySpacedRectSide\",\"uuid\":\"d9b66c7e-0954-4c47-8bcc-77bf13ff573c\"}]},\"type\":\"ConnectorPlacement.EquallySpacedConnector\",\"uuid\":\"345f3578-0572-4e64-b2f3-84728129a12d\"}],\"packageUris\":[\"http://schema.mathworks.com/mf0/Connector/R2020b\"],\"version\":\"1.0\"}"
  Vdcpr : Subsystem
      settings: PortSchema="{\"entries\":[{\"content\":{\"sides\":[{\"content\":{\"connectorIds\":[\"LConn1\",\"Out1\"]},\"type\":\"ConnectorPlacement.EquallySpacedRectSide\",\"uuid\":\"bc3757cc-4537-444e-89af-7b7d8c8c1fa7\"},{\"content\":{\"connectorIds\":[\"RConn1\"],\"side\":\"RIGHT\"},\"type\":\"ConnectorPlacement.EquallySpacedRectSide\",\"uuid\":\"908bf4c4-26f6-4d8a-bcf8-68236027f5f8\"},{\"content\":{\"side\":\"TOP\"},\"type\":\"ConnectorPlacement.EquallySpacedRectSide\",\"uuid\":\"33f228db-ba47-4718-96dc-a72de309ae8c\"},{\"content\":{\"side\":\"BOTTOM\"},\"type\":\"ConnectorPlacement.EquallySpacedRectSide\",\"uuid\":\"d9b66c7e-0954-4c47-8bcc-77bf13ff573c\"}]},\"type\":\"ConnectorPlacement.EquallySpacedConnector\",\"uuid\":\"345f3578-0572-4e64-b2f3-84728129a12d\"}],\"packageUris\":[\"http://schema.mathworks.com/mf0/Connector/R2020b\"],\"version\":\"1.0\"}"
  Vdcps : Subsystem
      settings: PortSchema="{\"entries\":[{\"content\":{\"sides\":[{\"content\":{\"connectorIds\":[\"LConn1\",\"Out1\"]},\"type\":\"ConnectorPlacement.EquallySpacedRectSide\",\"uuid\":\"bc3757cc-4537-444e-89af-7b7d8c8c1fa7\"},{\"content\":{\"connectorIds\":[\"RConn1\"],\"side\":\"RIGHT\"},\"type\":\"ConnectorPlacement.EquallySpacedRectSide\",\"uuid\":\"908bf4c4-26f6-4d8a-bcf8-68236027f5f8\"},{\"content\":{\"side\":\"TOP\"},\"type\":\"ConnectorPlacement.EquallySpacedRectSide\",\"uuid\":\"33f228db-ba47-4718-96dc-a72de309ae8c\"},{\"content\":{\"side\":\"BOTTOM\"},\"type\":\"ConnectorPlacement.EquallySpacedRectSide\",\"uuid\":\"d9b66c7e-0954-4c47-8bcc-77bf13ff573c\"}]},\"type\":\"ConnectorPlacement.EquallySpacedConnector\",\"uuid\":\"345f3578-0572-4e64-b2f3-84728129a12d\"}],\"packageUris\":[\"http://schema.mathworks.com/mf0/Connector/R2020b\"],\"version\":\"1.0\"}"
  P1 : PMIOPort  Side=Left
  N1 : PMIOPort  Port=2  Side=Left
  P2 : PMIOPort  Port=3  Side=Right
  N2 : PMIOPort  Port=4  Side=Right
  mDCS : Outport
  mDCR : Outport  Port=2
  wires:
  Vdcps/1(v) -> Bus Creator/1  "VdcpS"
  Vdcns/1(v) -> Bus Creator/2  "VdcnS"
  Idcps/1(i) -> Bus Creator/3  "IdcpS"
  Idcns/1(i) -> Bus Creator/4  "IdcnS"
  Bus Creator/1 -> mDCS/1
  Bus Creator1/1 -> mDCR/1
  Idcnr/1(i) -> Bus Creator1/4  "IdcnR"
  Idcpr/1(i) -> Bus Creator1/3  "IdcpR"
  Vdcpr/1(v) -> Bus Creator1/1  "VdcpR"
  Vdcnr/1(v) -> Bus Creator1/2  "VdcnR"
  connections:
  P1/RConn1 -- Idcps/LConn1 -- Cps/LConn1 -- Vdcps/LConn1
  Cns/RConn1 -- Idcns/LConn1 -- Vdcns/RConn1 -- N1/RConn1
  Vdcns/LConn1 -- Electrical Reference/LConn1 -- Cps/RConn1 -- Cns/LConn1 -- Vdcps/RConn1
  Negative Cable/LConn3 -- Electrical Reference3/LConn1 -- Negative Cable/LConn2
  Negative Cable/RConn3 -- Electrical Reference4/LConn1 -- Negative Cable/RConn2
  Positive Cable/LConn2 -- Electrical Reference1/LConn1 -- Positive Cable/LConn3
  Positive Cable/RConn3 -- Electrical Reference2/LConn1 -- Positive Cable/RConn2
  Idcpr/LConn1 -- Positive Cable/RConn1
  Idcnr/LConn1 -- Negative Cable/RConn1
  Positive Cable/LConn1 -- Idcps/RConn1
  Negative Cable/LConn1 -- Idcns/RConn1
  Cpr/RConn1 -- Vdcpr/RConn1 -- Vdcnr/LConn1 -- Electrical Reference5/LConn1 -- Cnr/LConn1
  Cnr/RConn1 -- N2/RConn1 -- Vdcnr/RConn1 -- Idcnr/RConn1
  Cpr/LConn1 -- Idcpr/RConn1 -- P2/RConn1 -- Vdcpr/LConn1

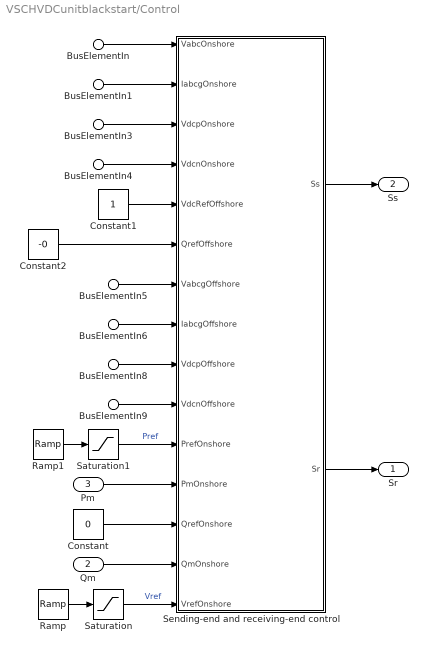
== system VSCHVDCunitblackstart/Control ==
  BusElementIn : Inport  PortName=mSEndAC  Element=vabcgS
  BusElementIn1 : Inport  PortName=mSEndAC  Element=iabcgS
  Qm : Inport  Port=2
  Pm : Inport  Port=3
  BusElementIn5 : Inport  Port=4  PortName=mREndAC  Element=signal1
  BusElementIn6 : Inport  Port=4  PortName=mREndAC  Element=signal2
  BusElementIn8 : Inport  Port=5  PortName=mREndDC  Element=VdcpR
  BusElementIn9 : Inport  Port=5  PortName=mREndDC  Element=VdcnR
  BusElementIn3 : Inport  Port=6  PortName=mSEndDC  Element=VdcpS
  BusElementIn4 : Inport  Port=6  PortName=mSEndDC  Element=VdcnS
  Constant : Constant  Value=0
  Constant1 : Constant
  Constant2 : Constant  Value=-0
  Ramp : simulink/Sources/Ramp  slope=0.5  start=20  InitialOutput=0
  Ramp1 : simulink/Sources/Ramp  slope=0.5  start=20  InitialOutput=0
  Saturation : Saturate  UpperLimit=1  LowerLimit=0
  Saturation1 : Saturate  UpperLimit=0.02  LowerLimit=0
  Sending-end and receiving-end control : Subsystem  mask{PRated=PRated, VRated=VRated*1.15, FRated=FRated, VdcRated=320e3, Nm=Nm, TranRL=[Rt Lt], ReRL=[Rr Lr], Rc=Rc, Ts=Ts*6, Tsc=Ts*6, InitUsingOP=off, Kq=-0.05, Kp=0.1, SEnd_P_PI=[0 19.2], SEnd_Q_PI=[0 18.9], SEnd_Id_PI=[0.61  12], SEnd_Iq_PI=[0.47  8.2], Vabcgs0=[-0.04077    -0.84632     0.88709], Vphases0=-0.040715, Vdqgs0=[1.0016           0], Iabcgs0=[0.16536    -0.77003     0.60466], Idqgs0=[0.78629     0.19753], P_PIs0=0.79269, Q_PIs0=0.1982, Id_PIs0=0.043811, Iq_PIs0=-0.086415, Vdcs0=401555.141, REnd_Vdc_PI=[1.8 12], REnd_Q_PI=[0 19], REnd_Id_PI=[0.76 13.4], REnd_Iq_PI=[0.58 9.5], Vabcgr0=[0.03658    -0.89332     0.85675], Vphaser0=0.036187, Vdqgr0=[1.0111           0], Iabcgr0=[0.070866     0.61731    -0.68817], Idqgr0=[-0.75066    0.098089], P_PIr0=-0.75404, Q_PIr0=0.098227, Id_PIr0=0.0050687, Iq_PIr0=0.086348, Vdcr0=400132.3608}
      mask prompts: PRated "Rated power (W)"; VRated "Rated AC voltage, rms line-to-line (V)"; FRated "Grid frequency (Hz)"; VdcRated "Rated DC voltage (V)"; Nm "Number of power submodules per arm"; TranRL "Transformer winding resistance and leakage inductance (pu)"; ReRL "Reactor resistance and inductance (pu)"; Rc "Equivalent cable resistance (Ohm)"; Ts "Fundamental sample time (s)"; Tsc "Control sample time (s)"; InitUsingOP "Initialize control using Simscape operating point"; Kq "Reactive Power Droop (pu)"; Kp "Active Power Droop (pu)"; SEnd_P_PI "Active power control proportional and integral gain"; SEnd_Q_PI "Reactive power control proportional and integral gain"; SEnd_Id_PI "D-axis current control proportional and integral gain"; SEnd_Iq_PI "Q-axis current control proportional and integral gain"; Vabcgs0 "Initial three-phase AC grid voltage (pu)"; Vphases0 "Initial phase angle of Phase-A voltage (rad)"; Vdqgs0 "Initial dq-axes grid voltage (pu)"; Iabcgs0 "Initial three-phase AC grid current (pu)"; Idqgs0 "Initial dq-axes grid current (pu)"; P_PIs0 "Initial state of active power PI (pu)"; Q_PIs0 "Initial state of reactive power PI (pu)"; Id_PIs0 "Initial state of d-axis current PI (pu)"; Iq_PIs0 "Initial state of q-axis current PI (pu)"; Vdcs0 "Initial sending-end DC voltage (V)"; REnd_Vdc_PI "DC voltage control proportional and integral gain"; REnd_Q_PI "Reactive power control proportional and integral gain"; REnd_Id_PI "D-axis current control proportional and integral gain"; REnd_Iq_PI "Q-axis current control proportional and integral gain"; Vabcgr0 "Initial three-phase AC grid voltage (pu)"; Vphaser0 "Initial phase angle of Phase-A voltage (rad)"; Vdqgr0 "Initial dq-axes grid voltage (pu)"; Iabcgr0 "Initial three-phase AC grid current (pu)"; Idqgr0 "Initial dq-axes grid current (pu)"; P_PIr0 "Initial state of DC voltage PI (pu)"; Q_PIr0 "Initial state of reactive power PI (pu)"; Id_PIr0 "Initial state of d-axis current PI (pu)"; Iq_PIr0 "Initial state of q-axis current PI (pu)"; Vdcr0 "Initial receiving-end DC voltage (V)"
      mask DialogControl Container4 Prompt: System
      mask DialogControl Container5 Prompt: Onshore Controller
      mask DialogControl Container6 Prompt: Offshore Controller
  Sr : Outport
  Ss : Outport  Port=2
  wires:
  BusElementIn/1 -> Sending-end and receiving-end control/1(VabcOnshore)
  BusElementIn1/1 -> Sending-end and receiving-end control/2(IabcgOnshore)
  BusElementIn3/1 -> Sending-end and receiving-end control/3(VdcpOnshore)
  BusElementIn4/1 -> Sending-end and receiving-end control/4(VdcnOnshore)
  Sending-end and receiving-end control/1(Ss) -> Ss/1
  Sending-end and receiving-end control/2(Sr) -> Sr/1
  BusElementIn8/1 -> Sending-end and receiving-end control/9(VdcpOffshore)
  BusElementIn9/1 -> Sending-end and receiving-end control/10(VdcnOffshore)
  BusElementIn6/1 -> Sending-end and receiving-end control/8(IabcgOffshore)
  BusElementIn5/1 -> Sending-end and receiving-end control/7(VabcgOffshore)
  Saturation1/1 -> Sending-end and receiving-end control/11(PrefOnshore)  "Pref"
  Pm/1 -> Sending-end and receiving-end control/12(PmOnshore)
  Qm/1 -> Sending-end and receiving-end control/14(QmOnshore)
  Constant/1 -> Sending-end and receiving-end control/13(QrefOnshore)
  Saturation/1 -> Sending-end and receiving-end control/15(VrefOnshore)  "Vref"
  Ramp/1 -> Saturation/1
  Ramp1/1 -> Saturation1/1
  Constant2/1 -> Sending-end and receiving-end control/6(QrefOffshore)
  Constant1/1 -> Sending-end and receiving-end control/5(VdcRefOffshore)

== system VSCHVDCunitblackstart/Offshore Station ==
  Reactor1 : ee_lib/Passive/RLC Assemblies/RLC (Three-Phase)  port_option=ee.enum.threePhasePort.composite  component_structure=ee.enum.rlc.structure.SeriesRL  R=Rr*Zbase Ohm  L=Lr*Lbase H  C=1e-6 F  R_parasitic=0 Ohm  G_parasitic=0 1/Ohm  IL_specify=off  IL_priority=High  IL=[0, 0, 0] A  IL_nominal_specify=off  IL_nominal_value=1  IL_nominal_unit=A  VC_specify=off  VC_priority=High  VC=[0, 0, 0] V  VC_nominal_specify=off  VC_nominal_value=1  VC_nominal_unit=V
      settings: InternalSimscapePortConfiguration="{\"Bottom\":[],\"Left\":[{\"id\":\"N1\",\"label\":\"~1\",\"type\":\"foundation.electrical.three_phase\"}],\"Right\":[{\"id\":\"N2\",\"label\":\"~2\",\"type\":\"foundation.electrical.three_phase\"}],\"Top\":[]}"
  Receiving-end vi : Subsystem
  Transformer : ee_lib/Passive/Transformers/Two-Winding Transformer (Three-Phase)  SRated=Pnom A*V  FRated=FRated Hz  Winding1Connection=ee.enum.windingconnection.Y  VRated1=Vt1 V  Winding2Connection=ee.enum.windingconnection.Y  VRated2=Vt2*1.15 V  CoreType=ee.enum.coretype.fivelimb  pu_Rw1=Rt/2  pu_Rw2=Rt/2  leakage_reactance_option=ee.enum.transformer_leakage.include  pu_Xl1=Lt/2  pu_Xl2=Lt/2  magnetizing_resistance_option=ee.enum.transformer_magnetizingResistance.include  pu_Rm=500  magnetizing_reactance_option=ee.enum.transformer_magnetizingReactance.include  saturation_option=ee.enum.transformer_saturation.exclude  pu_Xm=500  current_data=[0, .002, 1, 2]  magnetic_flux_data=[0, 1.2, 1.5, 1.51]  pu_X0=0.5  i1_specify=off  i1_priority=None  i1=[0, 0, 0] A  i1_nominal_specify=off  i1_nominal_value=1  i1_nominal_unit=A  i2_specify=off  i2_priority=None  i2=[0, 0, 0] A  i2_nominal_specify=off  i2_nominal_value=1  i2_nominal_unit=A  phi_specify=off  phi_priority=None  phi=[0, 0, 0]  phi_nominal_specify=off  phi_nominal_value=1  phi_nominal_unit=1  power_dissipated_specify=off  power_dissipated_priority=None  power_dissipated=0 W  power_dissipated_nominal_specify=off  power_dissipated_nominal_value=1  power_dissipated_nominal_unit=W
      settings: InternalSimscapePortConfiguration="{\"Bottom\":[],\"Left\":[{\"id\":\"N1\",\"label\":\"~1\",\"type\":\"foundation.electrical.three_phase\"}],\"Right\":[{\"id\":\"N2\",\"label\":\"~2\",\"type\":\"foundation.electrical.three_phase\"}],\"Top\":[]}"
      settings: AttributesFormatString=|
      | 400 MVA
      | 230 kV / 200 kV
  ~2 : PMIOPort  Side=Left
  Conn1 : PMIOPort  Port=2  Side=Right
  Out1 : Outport
  Out2 : Outport  Port=2
  wires:
  Receiving-end vi/1(v) -> Out2/1
  Receiving-end vi/2(i) -> Out1/1
  connections:
  Reactor1/LConn1 -- Transformer/RConn1
  Transformer/LConn1 -- Receiving-end vi/RConn1
  Conn1/RConn1 -- Reactor1/RConn1
  ~2/RConn1 -- Receiving-end vi/LConn1

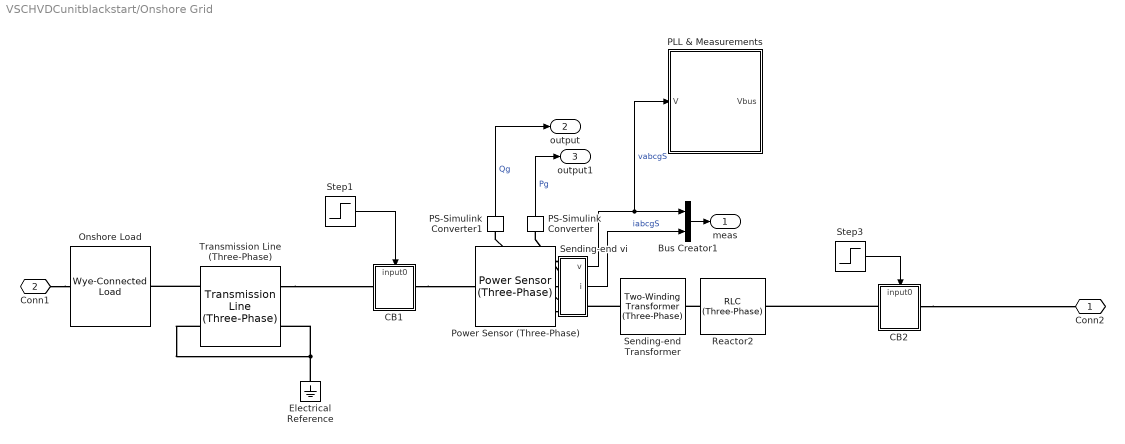
== system VSCHVDCunitblackstart/Onshore Grid ==
  Bus Creator1 : BusCreator  Inputs=2
  CB1 : Subsystem
      settings: PortSchema="{\"entries\":[{\"content\":{\"sides\":[{\"content\":{\"connectorIds\":[\"LConn1\"]},\"type\":\"ConnectorPlacement.EquallySpacedRectSide\",\"uuid\":\"67c0f727-7c15-41c9-98df-b3c7d57498ed\"},{\"content\":{\"connectorIds\":[\"RConn1\"],\"side\":\"RIGHT\"},\"type\":\"ConnectorPlacement.EquallySpacedRectSide\",\"uuid\":\"7fc39429-ba61-416d-b42b-93e81eb2f426\"},{\"content\":{\"side\":\"TOP\"},\"type\":\"ConnectorPlacement.EquallySpacedRectSide\",\"uuid\":\"c6dd9263-b57a-4cff-a218-af99f2798f29\"},{\"content\":{\"connectorIds\":[\"In1\"],\"side\":\"BOTTOM\"},\"type\":\"ConnectorPlacement.EquallySpacedRectSide\",\"uuid\":\"e2a2ba44-d59d-4e27-adf1-3f94e828ca78\"}]},\"type\":\"ConnectorPlacement.EquallySpacedConnector\",\"uuid\":\"b349a99b-c902-4df9-9c99-34841afb28dd\"}],\"packageUris\":[\"http://schema.mathworks.com/mf0/Connector/R2020b\"],\"version\":\"1.0\"}"
  CB2 : Subsystem
      settings: PortSchema="{\"entries\":[{\"content\":{\"sides\":[{\"content\":{\"connectorIds\":[\"LConn1\"]},\"type\":\"ConnectorPlacement.EquallySpacedRectSide\",\"uuid\":\"67c0f727-7c15-41c9-98df-b3c7d57498ed\"},{\"content\":{\"connectorIds\":[\"RConn1\"],\"side\":\"RIGHT\"},\"type\":\"ConnectorPlacement.EquallySpacedRectSide\",\"uuid\":\"7fc39429-ba61-416d-b42b-93e81eb2f426\"},{\"content\":{\"side\":\"TOP\"},\"type\":\"ConnectorPlacement.EquallySpacedRectSide\",\"uuid\":\"c6dd9263-b57a-4cff-a218-af99f2798f29\"},{\"content\":{\"connectorIds\":[\"In1\"],\"side\":\"BOTTOM\"},\"type\":\"ConnectorPlacement.EquallySpacedRectSide\",\"uuid\":\"e2a2ba44-d59d-4e27-adf1-3f94e828ca78\"}]},\"type\":\"ConnectorPlacement.EquallySpacedConnector\",\"uuid\":\"b349a99b-c902-4df9-9c99-34841afb28dd\"}],\"packageUris\":[\"http://schema.mathworks.com/mf0/Connector/R2020b\"],\"version\":\"1.0\"}"
  Electrical Reference : fl_lib/Electrical/Electrical Elements/Electrical Reference
  Onshore Load : ee_lib/Passive/RLC Assemblies/Wye-Connected Load  port_option=ee.enum.threePhasePort.composite  parameterization=ee.enum.rlc.parameterization.ratedpower  component_structure=ee.enum.rlc.structure.R  component_structure_PQ=ee.enum.rlc.structure.R  R=1 Ohm  L=1e-3 H  C=1e-6 F  VRated=VgridRated V  FRated=60 Hz  P=PRated*0.05 W  Qpos=1e2 A*V  Qneg=-1e2 A*V  R_parasitic=0 Ohm  G_parasitic=0 1/Ohm  R_parasitic_PQ=0 Ohm  G_parasitic_PQ=0 1/Ohm  Vmag0=24e3 V  Vang0=0 deg  Freq0=60 Hz  IL_specify=off  IL_priority=High  IL=[0, 0, 0] A  IL_nominal_specify=off  IL_nominal_value=1  IL_nominal_unit=A  VC_specify=off  VC_priority=High  VC=[0, 0, 0] V  VC_nominal_specify=off  VC_nominal_value=1  VC_nominal_unit=V
  PLL & Measurements : Subsystem
      settings: PortSchema="{\"entries\":[{\"content\":{\"sides\":[{\"content\":{\"connectorIds\":[\"Out1\"]},\"type\":\"ConnectorPlacement.EquallySpacedRectSide\",\"uuid\":\"76485780-20fe-4fcf-8224-69648da6ed2a\"},{\"content\":{\"connectorIds\":[\"In1\"],\"side\":\"RIGHT\"},\"type\":\"ConnectorPlacement.EquallySpacedRectSide\",\"uuid\":\"f19a6390-e634-42c7-8d46-4cd80cbab182\"},{\"content\":{\"side\":\"TOP\"},\"type\":\"ConnectorPlacement.EquallySpacedRectSide\",\"uuid\":\"87682f72-1844-428e-be70-ad7ca3191ee3\"}]},\"type\":\"ConnectorPlacement.EquallySpacedConnector\",\"uuid\":\"f2136b07-48ec-402b-adb3-18c0bac2157c\"}],\"packageUris\":[\"http://schema.mathworks.com/mf0/Connector/R2020b\"],\"version\":\"1.0\"}"
      mask Display: image('measurements.png'); % Use "Edit Image" on toolstrip to change.
  PS-Simulink Converter : nesl_utility/PS-Simulink Converter  PhysicalDomain=network_engine_domain  SubClassName=ps_output  LeftPortType=input  RightPortType=output  PseudoPeriodic=off  Frequencies=[]  VectorFormat=inherit  Unit=inherit  AffineConversion=off
  PS-Simulink Converter1 : nesl_utility/PS-Simulink Converter  PhysicalDomain=network_engine_domain  SubClassName=ps_output  LeftPortType=input  RightPortType=output  PseudoPeriodic=off  Frequencies=[]  VectorFormat=inherit  Unit=inherit  AffineConversion=off
  Power Sensor (Three-Phase) : ee_lib/Sensors & Transducers/Power Sensor (Three-Phase)  load_type=ee.enum.passive.type_balanced.balanced  f0=60 Hz
      settings: InternalSimscapePortConfiguration="{\"Bottom\":[],\"Left\":[{\"id\":\"N1\",\"label\":\"~1\",\"type\":\"foundation.electrical.three_phase\"}],\"Right\":[{\"id\":\"N2\",\"label\":\"~2\",\"type\":\"foundation.electrical.three_phase\"}],\"Top\":[{\"id\":\"Pm\",\"label\":\"P\",\"type\":\"output\"},{\"id\":\"Qm\",\"label\":\"Q\",\"type\":\"output\"}]}"
  Reactor2 : ee_lib/Passive/RLC Assemblies/RLC (Three-Phase)  port_option=ee.enum.threePhasePort.composite  component_structure=ee.enum.rlc.structure.SeriesRL  R=Rr*Zbase Ohm  L=Lr*Lbase H  C=1e-6 F  R_parasitic=0 Ohm  G_parasitic=0 1/Ohm  IL_specify=off  IL_priority=High  IL=[0, 0, 0] A  IL_nominal_specify=off  IL_nominal_value=1  IL_nominal_unit=A  VC_specify=off  VC_priority=High  VC=[0, 0, 0] V  VC_nominal_specify=off  VC_nominal_value=1  VC_nominal_unit=V
      settings: InternalSimscapePortConfiguration="{\"Bottom\":[],\"Left\":[{\"id\":\"N1\",\"label\":\"~1\",\"type\":\"foundation.electrical.three_phase\"}],\"Right\":[{\"id\":\"N2\",\"label\":\"~2\",\"type\":\"foundation.electrical.three_phase\"}],\"Top\":[]}"
  Sending-end Transformer : ee_lib/Passive/Transformers/Two-Winding Transformer (Three-Phase)  SRated=Pnom A*V  FRated=FRated Hz  Winding1Connection=ee.enum.windingconnection.Y  VRated1=Vt1 V  Winding2Connection=ee.enum.windingconnection.Yg  VRated2=Vt2*1.15 V  CoreType=ee.enum.coretype.fivelimb  pu_Rw1=Rt/2  pu_Rw2=Rt/2  leakage_reactance_option=ee.enum.transformer_leakage.include  pu_Xl1=Lt/2  pu_Xl2=Lt/2  magnetizing_resistance_option=ee.enum.transformer_magnetizingResistance.include  pu_Rm=500  magnetizing_reactance_option=ee.enum.transformer_magnetizingReactance.include  saturation_option=ee.enum.transformer_saturation.exclude  pu_Xm=500  current_data=[0, .002, 1, 2]  magnetic_flux_data=[0, 1.2, 1.5, 1.51]  pu_X0=0.5  i1_specify=off  i1_priority=High  i1=[0 0 0] A  i1_nominal_specify=off  i1_nominal_value=1  i1_nominal_unit=A  i2_specify=off  i2_priority=High  i2=[0 0 0] A  i2_nominal_specify=off  i2_nominal_value=1  i2_nominal_unit=A  phi_specify=off  phi_priority=None  phi=[0, 0, 0]  phi_nominal_specify=off  phi_nominal_value=1  phi_nominal_unit=1  power_dissipated_specify=off  power_dissipated_priority=None  power_dissipated=0 W  power_dissipated_nominal_specify=off  power_dissipated_nominal_value=1  power_dissipated_nominal_unit=W
      settings: InternalSimscapePortConfiguration="{\"Bottom\":[],\"Left\":[{\"id\":\"N1\",\"label\":\"~1\",\"type\":\"foundation.electrical.three_phase\"}],\"Right\":[{\"id\":\"N2\",\"label\":\"~2\",\"type\":\"foundation.electrical.three_phase\"}],\"Top\":[]}"
      settings: AttributesFormatString=|
      | 400 MVA
      | 230 kV / 200 kV
  Sending-end vi : Subsystem
  Step1 : Step  Time=20  Before=1  After=0  SampleTime=Ts
  Step3 : Step  Time=20  Before=1  After=0  SampleTime=Ts
  Transmission Line (Three-Phase) : ee_lib/Passive/Lines/Transmission Line (Three-Phase)  length=5 km  freq=60 Hz  R=0.02 Ohm/km  L=0.2 mH/km  M=0.01 mH/km  Cl=0.001 uF/km  Cg=0.1 uF/km  Rm=0 Ohm/km  ModelTwoSections=ee.enum.enable.no  N=1  InterfacePosition=0.5 km  N1sec=1  N2sec=1  Access_ground=ee.enum.enable.no  R_parasitic=1e-6 Ohm  G_parasitic=1e-6 1/Ohm
      settings: InternalSimscapePortConfiguration="{\"Bottom\":[],\"Left\":[{\"id\":\"N1\",\"label\":\"~1\",\"type\":\"foundation.electrical.three_phase\"},{\"id\":\"g1\",\"label\":\"g1\",\"type\":\"foundation.electrical.electrical\"}],\"Right\":[{\"id\":\"N2\",\"label\":\"~2\",\"type\":\"foundation.electrical.three_phase\"},{\"id\":\"g2\",\"label\":\"g2\",\"type\":\"foundation.electrical.electrical\"}],\"Top\":[]}"
  Conn2 : PMIOPort  Side=Right
  Conn1 : PMIOPort  Port=2  Side=Right
  meas : Outport
  output : Outport  Port=2
  output1 : Outport  Port=3
  wires:
  Sending-end vi/1(v) -> PLL & Measurements/1(V), Bus Creator1/1  "vabcgS"
  Bus Creator1/1 -> meas/1
  Sending-end vi/2(i) -> Bus Creator1/2  "iabcgS"
  PS-Simulink Converter/1 -> output1/1  "Pg"
  PS-Simulink Converter1/1 -> output/1  "Qg"
  Step3/1 -> CB2/1(input0)
  Step1/1 -> CB1/1(input0)
  connections:
  Power Sensor (Three-Phase)/LConn1 -- Sending-end vi/LConn1
  Sending-end Transformer/LConn1 -- Sending-end vi/RConn1
  Power Sensor (Three-Phase)/LConn3 -- PS-Simulink Converter1/LConn1
  Power Sensor (Three-Phase)/LConn2 -- PS-Simulink Converter/LConn1
  Reactor2/LConn1 -- Sending-end Transformer/RConn1
  Conn1/RConn1 -- Onshore Load/RConn1
  CB1/RConn1 -- Power Sensor (Three-Phase)/RConn1
  CB2/RConn1 -- Conn2/RConn1
  CB2/LConn1 -- Reactor2/RConn1
  Transmission Line (Three-Phase)/LConn1 -- Onshore Load/LConn1
  Transmission Line (Three-Phase)/RConn1 -- CB1/LConn1
  Electrical Reference/LConn1 -- Transmission Line (Three-Phase)/LConn2 -- Transmission Line (Three-Phase)/RConn2

== system VSCHVDCunitblackstart/PIR ==
  input0 : Inport
  Subsystem1 : Subsystem
      settings: PortSchema="{\"entries\":[{\"content\":{\"sides\":[{\"content\":{\"connectorIds\":[\"LConn1\",\"In1\"]},\"type\":\"ConnectorPlacement.EquallySpacedRectSide\",\"uuid\":\"4d523b2f-3490-490d-9193-0c3e52b1c3a1\"},{\"content\":{\"connectorIds\":[\"RConn1\"],\"side\":\"RIGHT\"},\"type\":\"ConnectorPlacement.EquallySpacedRectSide\",\"uuid\":\"1543a14a-65b5-4637-8d41-6da95a6ca307\"},{\"content\":{\"side\":\"TOP\"},\"type\":\"ConnectorPlacement.EquallySpacedRectSide\",\"uuid\":\"9fff8ee8-4727-466f-977a-681c4f14cc56\"}]},\"type\":\"ConnectorPlacement.EquallySpacedConnector\",\"uuid\":\"a46df766-bf17-4bd6-a8b3-579011040ee9\"}],\"packageUris\":[\"http://schema.mathworks.com/mf0/Connector/R2020b\"],\"version\":\"1.0\"}"
  Conn2 : PMIOPort  Side=Left
  Conn1 : PMIOPort  Port=2  Side=Right
  wires:
  input0/1 -> Subsystem1/1(input0)
  connections:
  Conn2/RConn1 -- Subsystem1/RConn1
  Subsystem1/LConn1 -- Conn1/RConn1
